simulink model "kalmanfilte_r14r"  (Simulink 7.0)
settings: Solver=FixedStepDiscrete  StartTime=0.0  StopTime=10.0  RelTol=1e-3
undefined symbols (not defined in the file): A, A1, B, B1, C, C1, D, D1, P1, Q, Q1, R, R1, x0, x1
settings Model: Creator=fo1521  LastModifiedBy=fo1521
settings DebuggingCC: SaveWithParameterizedLinksMsg=none  MultiTaskCondExecSysMsg=none  StrictBusMsg=None
settings HardwareCC: TargetHWDeviceType=32-bit Generic
settings RTWCC: IncludeERTFirstTime=on
settings GRTTargetCC: TargetFcnLib=ansi_tfl_tmw.mat

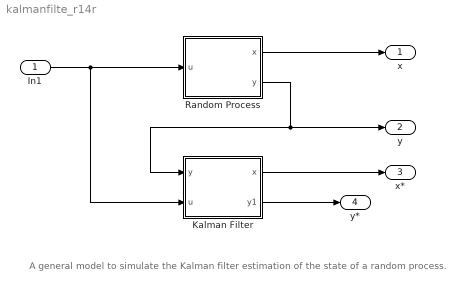
== system kalmanfilte_r14r ==
  note: A general model to simulate the Kalman filter estimation of the state of a random process.
  In1 : Inport  OutDataType=sfix(16)  OutScaling=2^0
  Kalman Filter : Subsystem  mask{x0=x1, P0=P1, A=A1, B=B1, C=C1, D=D1, Q=Q1, R=R1}
      mask help:
      | Linear Random Process
      | x(k+1)=Ax(k)+Bu(k)+w
      | y(k)=Cx(k)+Du(k)+v
      | w~N(0,Q)
      | w~N(0,R)
      mask Display:
      | disp(sprintf('Kalman\n Filter'))
      | port_label('output',2,'y')
      | port_label('output',1,'x')
      | port_label('input',1,'y')
      | port_label('input',2,'u')
  Random Process : Subsystem  mask{x0=x0, A=A, B=B, C=C, D=D, Q=sqrt(Q), R=sqrt(R)}
      mask help:
      | Linear Random Process
      | x(k+1)=Ax(k)+Bu(k)+w
      | y(k)=Cx(k)+Du(k)+v
      | w~N(0,Q)
      | w~N(0,R)
      mask Display:
      | disp(sprintf('Linear\n Random\n System'))
      | port_label('output',1,'x')
      | port_label('output',2,'y')
      | port_label('input',1,'u')
  x : Outport  OutDataType=sfix(16)  OutScaling=2^0
  y : Outport  Port=2  OutDataType=sfix(16)  OutScaling=2^0
  x* : Outport  Port=3  OutDataType=sfix(16)  OutScaling=2^0
  y* : Outport  Port=4  OutDataType=sfix(16)  OutScaling=2^0
  wires:
  Random Process/2(y) -> Kalman Filter/1(y), y/1
  In1/1 -> Random Process/1(u), Kalman Filter/2(u)
  Random Process/1(x) -> x/1
  Kalman Filter/1(x) -> x*/1
  Kalman Filter/2(y1) -> y*/1

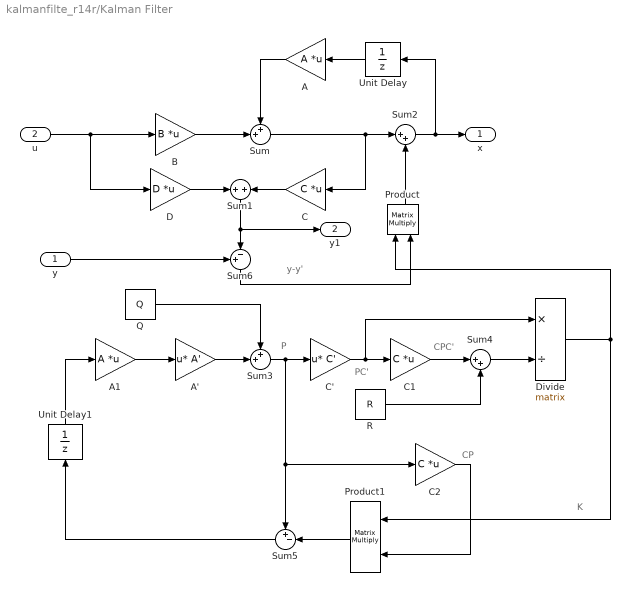
== system kalmanfilte_r14r/Kalman Filter ==
  note: P
  note: PC'
  note: CPC'
  note: K
  note: CP
  note: y-y'
  y : Inport  OutDataType=sfix(16)  OutScaling=2^0
  u : Inport  Port=2  PortDimensions=size(B,2)  OutDataType=sfix(16)  OutScaling=2^0
  A : Gain  Orientation=left  Gain=A  Multiplication=Matrix(K*u)  ParameterDataType=sfix(16)  ParameterScaling=2^0  OutDataType=sfix(16)  OutScaling=2^0
  A' : Gain  Gain=A'  Multiplication=Matrix(u*K)  ParameterDataType=sfix(16)  ParameterScaling=2^0  OutDataType=sfix(16)  OutScaling=2^0
  A1 : Gain  Gain=A  Multiplication=Matrix(K*u)  ParameterDataType=sfix(16)  ParameterScaling=2^0  OutDataType=sfix(16)  OutScaling=2^0
  B : Gain  Gain=B  Multiplication=Matrix(K*u)  ParameterDataType=sfix(16)  ParameterScaling=2^0  OutDataType=sfix(16)  OutScaling=2^0
  C : Gain  Orientation=left  Gain=C  Multiplication=Matrix(K*u)  ParameterDataType=sfix(16)  ParameterScaling=2^0  OutDataType=sfix(16)  OutScaling=2^0
  C' : Gain  Gain=C'  Multiplication=Matrix(u*K)  ParameterDataType=sfix(16)  ParameterScaling=2^0  OutDataType=sfix(16)  OutScaling=2^0
  C1 : Gain  Gain=C  Multiplication=Matrix(K*u)  ParameterDataType=sfix(16)  ParameterScaling=2^0  OutDataType=sfix(16)  OutScaling=2^0
  C2 : Gain  Gain=C  Multiplication=Matrix(K*u)  ParameterDataType=sfix(16)  ParameterScaling=2^0  OutDataType=sfix(16)  OutScaling=2^0
  D : Gain  Gain=D  Multiplication=Matrix(K*u)  ParameterDataType=sfix(16)  ParameterScaling=2^0  OutDataType=sfix(16)  OutScaling=2^0
  Divide : Product  Inputs=*/  Multiplication=Matrix(*)  OutDataType=sfix(16)  OutScaling=2^-10
  Product : Product  Orientation=up  Multiplication=Matrix(*)  OutDataType=sfix(16)  OutScaling=2^0  RndMeth=Zero
  Product1 : Product  Orientation=left  Multiplication=Matrix(*)  OutDataType=sfix(16)  OutScaling=2^0  RndMeth=Zero
  Q : Constant  Value=Q  OutDataType=sfix(16)  OutScaling=2^0
  R : Constant  Value=R  OutDataType=sfix(16)  OutScaling=2^0
  Sum : Sum  Inputs=++|  OutDataType=sfix(16)  OutScaling=2^0
  Sum1 : Sum  Orientation=down  Inputs=+|+  OutDataType=sfix(16)  OutScaling=2^0
  Sum2 : Sum  Inputs=|++  OutDataType=sfix(16)  OutScaling=2^0
  Sum3 : Sum  Inputs=++|  OutDataType=sfix(16)  OutScaling=2^0
  Sum4 : Sum  Inputs=|++  OutDataType=sfix(16)  OutScaling=2^0
  Sum5 : Sum  Orientation=left  Inputs=+-|  OutDataType=sfix(16)  OutScaling=2^0
  Sum6 : Sum  Orientation=down  Inputs=+-|  OutDataType=sfix(16)  OutScaling=2^0
  Unit Delay : UnitDelay  Orientation=left  X0=x0
  Unit Delay1 : UnitDelay  Orientation=up  X0=P0
  x : Outport  OutDataType=sfix(16)  OutScaling=2^0
  y1 : Outport  Port=2  OutDataType=sfix(16)  OutScaling=2^0
  wires:
  u/1 -> B/1, D/1
  B/1 -> Sum/2
  A/1 -> Sum/1
  Unit Delay/1 -> A/1
  Sum/1 -> Sum2/1, C/1
  Sum2/1 -> x/1, Unit Delay/1
  D/1 -> Sum1/1
  C/1 -> Sum1/2
  A1/1 -> A'/1
  A'/1 -> Sum3/2
  Q/1 -> Sum3/1
  Sum3/1 -> C'/1, Sum5/1, C2/1
  C'/1 -> C1/1, Divide/1
  Product/1 -> Sum2/2
  Divide/1 -> Product/1, Product1/1
  Product1/1 -> Sum5/2
  C1/1 -> Sum4/1
  R/1 -> Sum4/2
  Sum4/1 -> Divide/2
  Unit Delay1/1 -> A1/1
  Sum5/1 -> Unit Delay1/1
  C2/1 -> Product1/2
  Sum1/1 -> Sum6/2, y1/1
  y/1 -> Sum6/1
  Sum6/1 -> Product/2

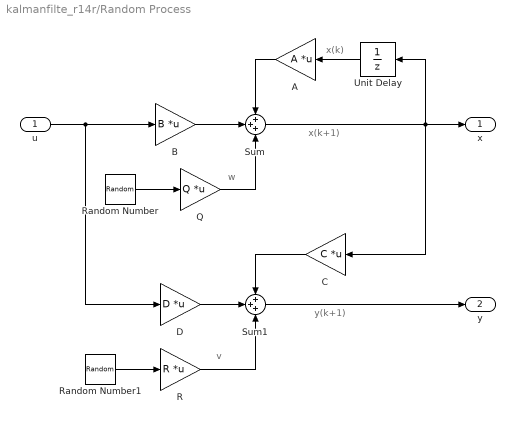
== system kalmanfilte_r14r/Random Process ==
  note: x(k+1)
  note: y(k+1)
  note: x(k)
  note: w
  note: v
  u : Inport  PortDimensions=size(B,2)  OutDataType=sfix(16)  OutScaling=2^0
  A : Gain  Orientation=left  Gain=A  Multiplication=Matrix(K*u)  ParameterDataType=sfix(16)  ParameterScaling=2^0  OutDataType=sfix(16)  OutScaling=2^0
  B : Gain  Gain=B  Multiplication=Matrix(K*u)  ParameterDataType=sfix(16)  ParameterScaling=2^0  OutDataType=sfix(16)  OutScaling=2^0
  C : Gain  Orientation=left  Gain=C  Multiplication=Matrix(K*u)  ParameterDataType=sfix(16)  ParameterScaling=2^0  OutDataType=sfix(16)  OutScaling=2^0
  D : Gain  Gain=D  Multiplication=Matrix(K*u)  ParameterDataType=sfix(16)  ParameterScaling=2^0  OutDataType=sfix(16)  OutScaling=2^0
  Q : Gain  Gain=Q  Multiplication=Matrix(K*u)  ParameterDataType=sfix(16)  ParameterScaling=2^0  OutDataType=sfix(16)  OutScaling=2^0
  R : Gain  Gain=R  Multiplication=Matrix(K*u)  ParameterDataType=sfix(16)  ParameterScaling=2^0  OutDataType=sfix(16)  OutScaling=2^0
  Random Number : RandomNumber  Mean=zeros(size(Q,1),1)  Variance=ones(size(Q,1),1)  Seed=7  SampleTime=1
  Random Number1 : RandomNumber  Mean=zeros(size(R,1),1)  Variance=ones(size(R,1),1)  SampleTime=1
  Sum : Sum  Inputs=+++  OutDataType=sfix(16)  OutScaling=2^0
  Sum1 : Sum  Inputs=+++  OutDataType=sfix(16)  OutScaling=2^0
  Unit Delay : UnitDelay  Orientation=left  X0=x0
  x : Outport  OutDataType=sfix(16)  OutScaling=2^0
  y : Outport  Port=2  OutDataType=sfix(16)  OutScaling=2^0
  wires:
  u/1 -> B/1, D/1
  Random Number/1 -> Q/1
  B/1 -> Sum/2
  C/1 -> Sum1/1
  D/1 -> Sum1/2
  Random Number1/1 -> R/1
  R/1 -> Sum1/3
  Sum1/1 -> y/1
  Sum/1 -> Unit Delay/1, x/1, C/1
  Unit Delay/1 -> A/1
  A/1 -> Sum/1
  Q/1 -> Sum/3
